simulink model "Lesson2NVDHDongCo"  (R2014a)
settings: Solver=ode45  StartTime=0.0  StopTime=10.0  RelTol=1e-3
settings Model: Creator=tri  LastModifiedBy=tri

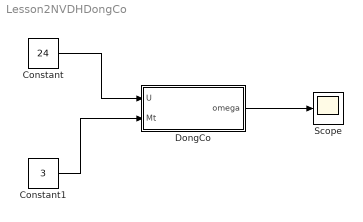
== system Lesson2NVDHDongCo ==
  Constant : Constant  Value=24
  Constant1 : Constant  Value=3
  DongCo : Subsystem  mask{Ru=1, phi=1, K=1, Tc=0.4, B=0.01, Tu=0.4}
      mask prompts: Ru "dien tro phan ung dong co"; phi "tu thong kich tu"; K "he so K"; Tc "thoi gian dien co"; B "he so ma sat"; Tu "thoi gian dien tu"
  Scope : Scope
  wires:
  Constant/1 -> DongCo/1(U)
  Constant1/1 -> DongCo/2(Mt)
  DongCo/1(omega) -> Scope/1

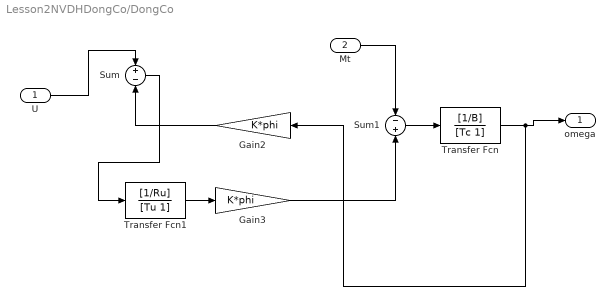
== system Lesson2NVDHDongCo/DongCo ==
  U : Inport
  Mt : Inport  Port=2
  Gain2 : Gain  Gain=K*phi
  "Gain3 " : Gain  Gain=K*phi
  Sum : Sum  Inputs=+-
  Sum1 : Sum  Inputs=-+
  Transfer Fcn : TransferFcn  Numerator=[1/B]  Denominator=[Tc 1]
  Transfer Fcn1 : TransferFcn  Numerator=[1/Ru]  Denominator=[Tu 1]
  omega : Outport
  wires:
  U/1 -> Sum/1
  Gain2/1 -> Sum/2
  Sum1/1 -> Transfer Fcn/1
  Mt/1 -> Sum1/1
  Transfer Fcn/1 -> Gain2/1, omega/1
  "Gain3 "/1 -> Sum1/2
  Transfer Fcn1/1 -> "Gain3 "/1
  Sum/1 -> Transfer Fcn1/1
